simulink model "FinalProjectSimulinkModel_OBSTACLE"  (R2023b)
settings: Solver=VariableStepAuto  StartTime=0.0  StopTime=17  RelTol=1e-3
values from neighbouring files (symbols this model uses):
  dq_d_COM = [0.75; 0; 0; 0; 0; 0]    [FinalProject_init.m]
  dq_d_COM_Jump = [10; 0; 20; 0; -30; 0]    [FinalProject_init.m]
  dq_d_COM_Jump_2 = [12; 0; 21.2; 0; -35.6; 0]    [FinalProject_init.m]
  dtMPC = 0.03    [FinalProject_init.m]
  firstStairDist = 0.26    [FinalProject_init.m]
  flight_gait_2 = [tcrouch2;fFofft2;rFofft2;rlandt2;flandt2; tImpact]    [FinalProject_init.m]
  flight_gait_t = [tcrouch;fFofft;rFofft;rlandt;flandt; tImpact]    [FinalProject_init.m]
  kd_swing = 10    [FinalProject_init.m]
  kp_swing = 300    [FinalProject_init.m]
  kStep = 0.001    [FinalProject_init.m]
  NMPC = 10    [FinalProject_init.m]
  offsets = [0;tSwing;tSwing;0]    [FinalProject_init.m]
  q_d_crouch = [q_hip_roll_f ... (first row only)    [FinalProject_init.m]
  q_d_impact = [q_hip_roll_i_f ... (first row only)    [FinalProject_init.m]
  q_d_stand = [q_hip_roll_i;q_hip_pitch_i;q_knee_i]    [FinalProject_init.m]
  q_hip_roll_i = 0    [FinalProject_init.m]
  Qmpc = diag([100 100 50 1000 1000 500 4 4 4 1 1 1 0])    [FinalProject_init.m]
  rFofft = 0.12+tcrouch    (= 1.12)    [FinalProject_init.m]
  rFofft2 = 0.12+tcrouch2    (= 1.42)    [FinalProject_init.m]
  Rmpc = 0.00001*eye(12)    [FinalProject_init.m]
  task = 6    [FinalProject_init.m]
  tcrouch = 1.0    (= 1)    [FinalProject_init.m]
  tcrouch2 = 1.3    [FinalProject_init.m]
  tCycle = 0.3    [FinalProject_init.m]
  tRamp = 0.5    [FinalProject_init.m]
  tRamp_Jump = 0.05    [FinalProject_init.m]
  tRamp_Jump2 = 0.08    [FinalProject_init.m]
  tSlow = 0.3    [FinalProject_init.m]
  tSwing = tCycle/2    (= 0.15)    [FinalProject_init.m]
  x0_Trunk = [0;0;z_trunk_i-.15; 0;-0.271;0]    [FinalProject_init.m]
undefined symbols (not defined in the file or in its folder): kStepTheta, X, Y, Z
libraries: sm_lib x199, nesl_utility x53
(part 2 of 6)

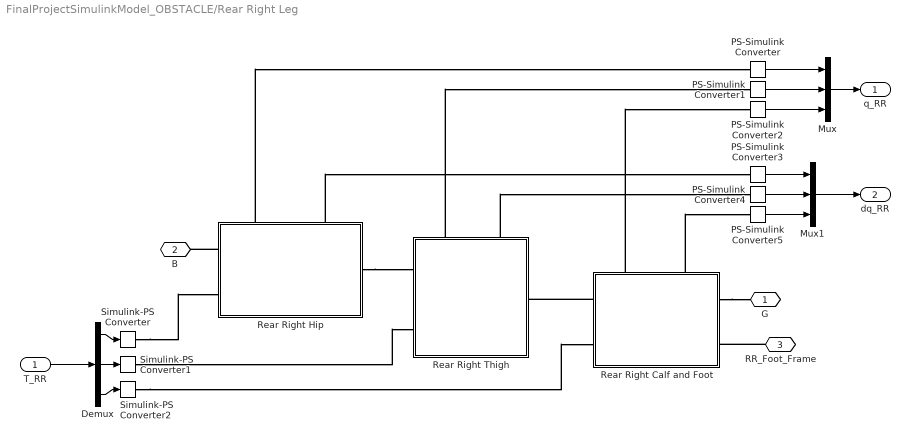
== system FinalProjectSimulinkModel_OBSTACLE/Rear Right Leg ==
  T_RR : Inport
  Demux : Demux  Outputs=3
  Mux : Mux  Inputs=3
  Mux1 : Mux  Inputs=3
  PS-Simulink Converter{,1..5} (6 alike) : nesl_utility/PS-Simulink Converter  PhysicalDomain=network_engine_domain  SubClassName=ps_output  LeftPortType=input  RightPortType=output  PseudoPeriodic=off  Frequencies=[]  VectorFormat=inherit  Unit=inherit  AffineConversion=off
  Rear Right Hip : Subsystem
      settings: PortSchema="{\"entries\":[{\"content\":{\"sides\":[{\"content\":{\"connectorIds\":[\"LConn1\",\"LConn2\"]},\"type\":\"ConnectorPlacement.EquallySpacedRectSide\",\"uuid\":\"d53fc21f-a4e5-460f-be2d-383a76a109ad\"},{\"content\":{\"connectorIds\":[\"RConn1\"],\"side\":\"RIGHT\"},\"type\":\"ConnectorPlacement.EquallySpacedRectSide\",\"uuid\":\"4a22f7e2-1f22-4597-903e-3f257006dede\"},{\"content\":{\"connectorIds\":[\"LConn3\",\"LConn4\"],\"side\":\"TOP\"},\"type\":\"ConnectorPlacement.EquallySpacedRectSide\",\"uuid\":\"7ea439a1-197b-4788-b0d2-cace68ebb6cf\"}]},\"type\":\"ConnectorPlacement.EquallySpacedConnector\",\"uuid\":\"bb801113-64bf-4d16-9167-4042132993b1\"}],\"packageUris\":[\"http://schema.mathworks.com/mf0/Connector/R2020b\"],\"version\":\"1.0\"}"
  Rear Right Thigh : Subsystem
      settings: PortSchema="{\"entries\":[{\"content\":{\"sides\":[{\"content\":{\"connectorIds\":[\"LConn1\",\"LConn2\"]},\"type\":\"ConnectorPlacement.EquallySpacedRectSide\",\"uuid\":\"d53fc21f-a4e5-460f-be2d-383a76a109ad\"},{\"content\":{\"connectorIds\":[\"RConn1\"],\"side\":\"RIGHT\"},\"type\":\"ConnectorPlacement.EquallySpacedRectSide\",\"uuid\":\"4a22f7e2-1f22-4597-903e-3f257006dede\"},{\"content\":{\"connectorIds\":[\"LConn3\",\"LConn4\"],\"side\":\"TOP\"},\"type\":\"ConnectorPlacement.EquallySpacedRectSide\",\"uuid\":\"7ea439a1-197b-4788-b0d2-cace68ebb6cf\"}]},\"type\":\"ConnectorPlacement.EquallySpacedConnector\",\"uuid\":\"bb801113-64bf-4d16-9167-4042132993b1\"}],\"packageUris\":[\"http://schema.mathworks.com/mf0/Connector/R2020b\"],\"version\":\"1.0\"}"
  Rear Right Calf and Foot : Subsystem
      settings: PortSchema="{\"entries\":[{\"content\":{\"sides\":[{\"content\":{\"connectorIds\":[\"LConn1\",\"LConn2\"]},\"type\":\"ConnectorPlacement.EquallySpacedRectSide\",\"uuid\":\"d53fc21f-a4e5-460f-be2d-383a76a109ad\"},{\"content\":{\"connectorIds\":[\"RConn1\",\"RConn2\"],\"side\":\"RIGHT\"},\"type\":\"ConnectorPlacement.EquallySpacedRectSide\",\"uuid\":\"4a22f7e2-1f22-4597-903e-3f257006dede\"},{\"content\":{\"connectorIds\":[\"LConn3\",\"LConn4\"],\"side\":\"TOP\"},\"type\":\"ConnectorPlacement.EquallySpacedRectSide\",\"uuid\":\"7ea439a1-197b-4788-b0d2-cace68ebb6cf\"}]},\"type\":\"ConnectorPlacement.EquallySpacedConnector\",\"uuid\":\"bb801113-64bf-4d16-9167-4042132993b1\"}],\"packageUris\":[\"http://schema.mathworks.com/mf0/Connector/R2020b\"],\"version\":\"1.0\"}"
  Simulink-PS Converter : nesl_utility/Simulink-PS Converter  PhysicalDomain=network_engine_domain  SubClassName=ps_input  LeftPortType=input  RightPortType=output  PseudoPeriodic=off  Frequencies=[]  NoiseDistribution=none  NoiseParameters=[]  Unit=1  AffineConversion=off  FilteringAndDerivatives=provide  SimscapeFilterOrder=1  InputFilterTimeConstant=0.001  UdotUserProvided=0
  Simulink-PS Converter1 : nesl_utility/Simulink-PS Converter  PhysicalDomain=network_engine_domain  SubClassName=ps_input  LeftPortType=input  RightPortType=output  PseudoPeriodic=off  Frequencies=[]  NoiseDistribution=none  NoiseParameters=[]  Unit=1  AffineConversion=off  FilteringAndDerivatives=provide  SimscapeFilterOrder=1  InputFilterTimeConstant=0.001  UdotUserProvided=0
  Simulink-PS Converter2 : nesl_utility/Simulink-PS Converter  PhysicalDomain=network_engine_domain  SubClassName=ps_input  LeftPortType=input  RightPortType=output  PseudoPeriodic=off  Frequencies=[]  NoiseDistribution=none  NoiseParameters=[]  Unit=1  AffineConversion=off  FilteringAndDerivatives=provide  SimscapeFilterOrder=1  InputFilterTimeConstant=0.001  UdotUserProvided=0
  G : PMIOPort  Side=Right
  B : PMIOPort  Port=2  Side=Left
  RR_Foot_Frame : PMIOPort  Port=3  Side=Right
  q_RR : Outport
  dq_RR : Outport  Port=2
  wires:
  T_RR/1 -> Demux/1
  Demux/2 -> Simulink-PS Converter1/1
  Demux/1 -> Simulink-PS Converter/1
  Demux/3 -> Simulink-PS Converter2/1
  PS-Simulink Converter/1 -> Mux/1
  PS-Simulink Converter1/1 -> Mux/2
  PS-Simulink Converter2/1 -> Mux/3
  PS-Simulink Converter4/1 -> Mux1/2
  PS-Simulink Converter5/1 -> Mux1/3
  PS-Simulink Converter3/1 -> Mux1/1
  Mux/1 -> q_RR/1
  Mux1/1 -> dq_RR/1
  connections:
  Rear Right Calf and Foot/LConn1 -- Rear Right Thigh/RConn1
  Rear Right Hip/RConn1 -- Rear Right Thigh/LConn1
  Rear Right Calf and Foot/RConn1 -- G/RConn1
  Rear Right Hip/LConn1 -- B/RConn1
  Simulink-PS Converter/RConn1 -- Rear Right Hip/LConn2
  Simulink-PS Converter1/RConn1 -- Rear Right Thigh/LConn2
  Simulink-PS Converter2/RConn1 -- Rear Right Calf and Foot/LConn2
  Rear Right Hip/LConn3 -- PS-Simulink Converter/LConn1
  Rear Right Thigh/LConn3 -- PS-Simulink Converter1/LConn1
  Rear Right Calf and Foot/LConn3 -- PS-Simulink Converter2/LConn1
  Rear Right Hip/LConn4 -- PS-Simulink Converter3/LConn1
  Rear Right Thigh/LConn4 -- PS-Simulink Converter4/LConn1
  Rear Right Calf and Foot/LConn4 -- PS-Simulink Converter5/LConn1
  RR_Foot_Frame/RConn1 -- Rear Right Calf and Foot/RConn2

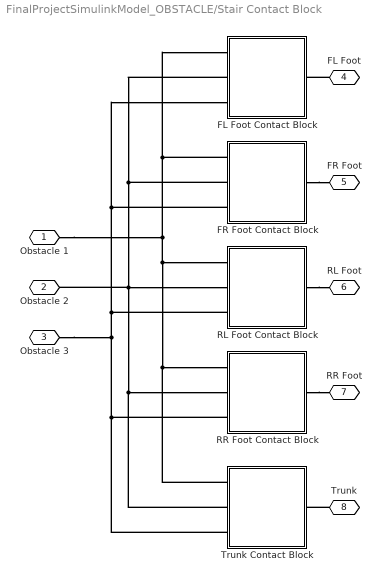
== system FinalProjectSimulinkModel_OBSTACLE/Stair Contact Block ==
  FL Foot Contact Block : Subsystem
  FR Foot Contact Block : Subsystem
  RL Foot Contact Block : Subsystem
  RR Foot Contact Block : Subsystem
  Trunk Contact Block : Subsystem
  Obstacle 1 : PMIOPort  Side=Left
  Obstacle 2 : PMIOPort  Port=2  Side=Left
  Obstacle 3 : PMIOPort  Port=3  Side=Left
  FL Foot : PMIOPort  Port=4  Side=Right
  FR Foot : PMIOPort  Port=5  Side=Right
  RL Foot : PMIOPort  Port=6  Side=Right
  RR Foot : PMIOPort  Port=7  Side=Right
  Trunk : PMIOPort  Port=8  Side=Right
  connections:
  Obstacle 1/RConn1 -- Trunk Contact Block/LConn1 -- RR Foot Contact Block/LConn1 -- RL Foot Contact Block/LConn1 -- FR Foot Contact Block/LConn1 -- FL Foot Contact Block/LConn1
  FL Foot Contact Block/LConn2 -- FR Foot Contact Block/LConn2 -- Trunk Contact Block/LConn2 -- RR Foot Contact Block/LConn2 -- Obstacle 2/RConn1 -- RL Foot Contact Block/LConn2
  Obstacle 3/RConn1 -- FR Foot Contact Block/LConn3 -- FL Foot Contact Block/LConn3 -- RL Foot Contact Block/LConn3 -- Trunk Contact Block/LConn3 -- RR Foot Contact Block/LConn3
  FR Foot Contact Block/RConn1 -- FR Foot/RConn1
  FL Foot/RConn1 -- FL Foot Contact Block/RConn1
  RL Foot Contact Block/RConn1 -- RL Foot/RConn1
  RR Foot Contact Block/RConn1 -- RR Foot/RConn1
  Trunk/RConn1 -- Trunk Contact Block/RConn1

== system FinalProjectSimulinkModel_OBSTACLE/base ==
  ReferenceFrame : sm_lib/Frames and Transforms/Reference Frame
  Visual : sm_lib/Body Elements/Brick Solid  GraphicAmbientColor=[0.15 0.15 0.15 1.0]  BasedOnType=Density  BrickDimensions=[0.001, 0.001, 0.001]  BrickDimensionsUnits=m  CenterOfMass=[0, 0, 0]  CenterOfMassUnits=m  GraphicDiffuseColor=[0.5, 0.5, 0.5]  Density=1000  DensityUnits=kg/m^3  DoExposeReferenceFrame=on  GraphicEmissiveColor=[0.0 0.0 0.0 1.0]  ExportEntireGeometry=off  SerializedFrames=<Frames/>  MarkerShape=Sphere  MarkerSize=10  GraphicType=FromGeometry  InertiaType=Custom  Mass=0  MassUnits=kg  MomentsOfInertia=[0, 0, 0]  MomentsOfInertiaUnits=kg*m^2  GraphicOpacity=1  ProductsOfInertia=[0, 0, 0]  ProductsOfInertiaUnits=kg*m^2  GraphicShininess=75  GraphicSpecularColor=[0.5 0.5 0.5 1.0]  GraphicVisPropType=SimpleVisualProperties
  VisualOriginTransform : sm_lib/Frames and Transforms/Rigid Transform  TranslationMethod=Cartesian  TranslationStandardOffset=0  TranslationStandardOffsetUnits=m  TranslationStandardAxis=+Z  TranslationCartesianOffset=[0, 0, 0]  TranslationCartesianOffsetUnits=m  TranslationROffset=0  TranslationROffsetUnits=m  TranslationZOffset=0  TranslationZOffsetUnits=m  TranslationThetaOffset=0  TranslationThetaOffsetUnits=deg  RotationMethod=RotationSequence  RotationAngleUnits=deg  RotationStandardAxis=+Z  RotationAngle=0.0  RotationArbitraryAxis=[0 0 1]  FollAlignAxisA=+X  BaseAlignAxisA=+Y  FollAlignAxisB=+Y  BaseAlignAxisB=+Z  RotationSequenceAxes=BaseAxes  RotationSequence=XYZ  RotationSequenceAngles=[0, 0, 0]  RotationSequenceAnglesUnits=rad  RotationMatrix=[1 0 0; 0 1 0; 0 0 1]  Quaternion=[1 0 0 0]
  floating_base_OriginTransform : sm_lib/Frames and Transforms/Rigid Transform  TranslationMethod=Cartesian  TranslationStandardOffset=0  TranslationStandardOffsetUnits=m  TranslationStandardAxis=+Z  TranslationCartesianOffset=[0, 0, 0]  TranslationCartesianOffsetUnits=m  TranslationROffset=0  TranslationROffsetUnits=m  TranslationZOffset=0  TranslationZOffsetUnits=m  TranslationThetaOffset=0  TranslationThetaOffsetUnits=deg  RotationMethod=RotationSequence  RotationAngleUnits=deg  RotationStandardAxis=+Z  RotationAngle=0.0  RotationArbitraryAxis=[0 0 1]  FollAlignAxisA=+X  BaseAlignAxisA=+Y  FollAlignAxisB=+Y  BaseAlignAxisB=+Z  RotationSequenceAxes=BaseAxes  RotationSequence=XYZ  RotationSequenceAngles=[0, 0, 0]  RotationSequenceAnglesUnits=rad  RotationMatrix=[1 0 0; 0 1 0; 0 0 1]  Quaternion=[1 0 0 0]
  F : PMIOPort  Side=Left
  F1 : PMIOPort  Port=2  Side=Right
  connections:
  VisualOriginTransform/LConn1 -- ReferenceFrame/RConn1 -- F/RConn1 -- floating_base_OriginTransform/LConn1
  Visual/RConn1 -- VisualOriginTransform/RConn1
  floating_base_OriginTransform/RConn1 -- F1/RConn1

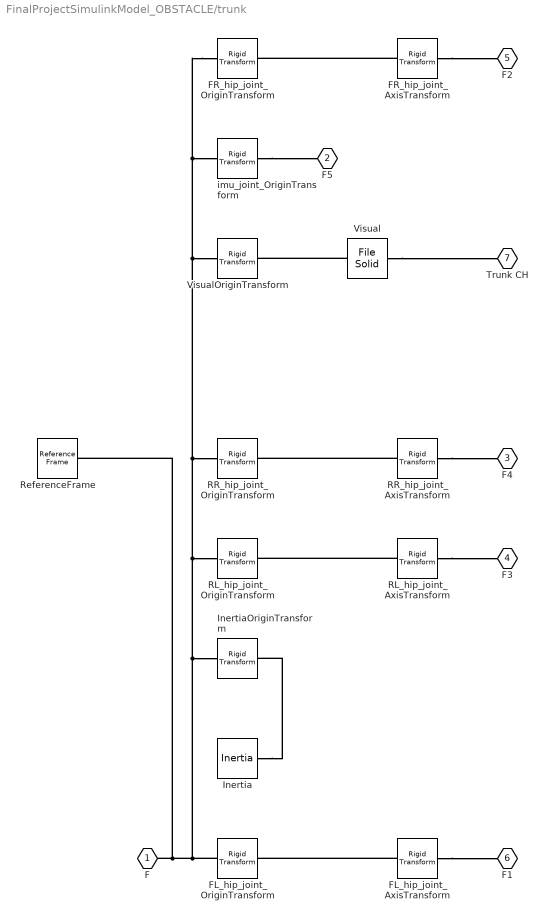
== system FinalProjectSimulinkModel_OBSTACLE/trunk ==
  FL_hip_joint_AxisTransform : sm_lib/Frames and Transforms/Rigid Transform  TranslationMethod=Cartesian  TranslationStandardOffset=0  TranslationStandardOffsetUnits=m  TranslationStandardAxis=+Z  TranslationCartesianOffset=[0, 0, 0]  TranslationCartesianOffsetUnits=m  TranslationROffset=0  TranslationROffsetUnits=m  TranslationZOffset=0  TranslationZOffsetUnits=m  TranslationThetaOffset=0  TranslationThetaOffsetUnits=deg  RotationMethod=ArbitraryAxis  RotationAngleUnits=rad  RotationStandardAxis=+Z  RotationAngle=1.570796326794897  RotationArbitraryAxis=[-0, 1, 0]  FollAlignAxisA=+X  BaseAlignAxisA=+Y  FollAlignAxisB=+Y  BaseAlignAxisB=+Z  RotationSequenceAxes=FollowerAxes  RotationSequence=XYX  RotationSequenceAngles=[0 0 0]  RotationSequenceAnglesUnits=deg  RotationMatrix=[1 0 0; 0 1 0; 0 0 1]  Quaternion=[1 0 0 0]
  FL_hip_joint_OriginTransform : sm_lib/Frames and Transforms/Rigid Transform  TranslationMethod=Cartesian  TranslationStandardOffset=0  TranslationStandardOffsetUnits=m  TranslationStandardAxis=+Z  TranslationCartesianOffset=[0.1805, 0.047, 0]  TranslationCartesianOffsetUnits=m  TranslationROffset=0  TranslationROffsetUnits=m  TranslationZOffset=0  TranslationZOffsetUnits=m  TranslationThetaOffset=0  TranslationThetaOffsetUnits=deg  RotationMethod=RotationSequence  RotationAngleUnits=deg  RotationStandardAxis=+Z  RotationAngle=0.0  RotationArbitraryAxis=[0 0 1]  FollAlignAxisA=+X  BaseAlignAxisA=+Y  FollAlignAxisB=+Y  BaseAlignAxisB=+Z  RotationSequenceAxes=BaseAxes  RotationSequence=XYZ  RotationSequenceAngles=[0, 0, 0]  RotationSequenceAnglesUnits=rad  RotationMatrix=[1 0 0; 0 1 0; 0 0 1]  Quaternion=[1 0 0 0]
  FR_hip_joint_AxisTransform : sm_lib/Frames and Transforms/Rigid Transform  TranslationMethod=Cartesian  TranslationStandardOffset=0  TranslationStandardOffsetUnits=m  TranslationStandardAxis=+Z  TranslationCartesianOffset=[0, 0, 0]  TranslationCartesianOffsetUnits=m  TranslationROffset=0  TranslationROffsetUnits=m  TranslationZOffset=0  TranslationZOffsetUnits=m  TranslationThetaOffset=0  TranslationThetaOffsetUnits=deg  RotationMethod=ArbitraryAxis  RotationAngleUnits=rad  RotationStandardAxis=+Z  RotationAngle=1.570796326794897  RotationArbitraryAxis=[-0, 1, 0]  FollAlignAxisA=+X  BaseAlignAxisA=+Y  FollAlignAxisB=+Y  BaseAlignAxisB=+Z  RotationSequenceAxes=FollowerAxes  RotationSequence=XYX  RotationSequenceAngles=[0 0 0]  RotationSequenceAnglesUnits=deg  RotationMatrix=[1 0 0; 0 1 0; 0 0 1]  Quaternion=[1 0 0 0]
  FR_hip_joint_OriginTransform : sm_lib/Frames and Transforms/Rigid Transform  TranslationMethod=Cartesian  TranslationStandardOffset=0  TranslationStandardOffsetUnits=m  TranslationStandardAxis=+Z  TranslationCartesianOffset=[0.1805, -0.047, 0]  TranslationCartesianOffsetUnits=m  TranslationROffset=0  TranslationROffsetUnits=m  TranslationZOffset=0  TranslationZOffsetUnits=m  TranslationThetaOffset=0  TranslationThetaOffsetUnits=deg  RotationMethod=RotationSequence  RotationAngleUnits=deg  RotationStandardAxis=+Z  RotationAngle=0.0  RotationArbitraryAxis=[0 0 1]  FollAlignAxisA=+X  BaseAlignAxisA=+Y  FollAlignAxisB=+Y  BaseAlignAxisB=+Z  RotationSequenceAxes=BaseAxes  RotationSequence=XYZ  RotationSequenceAngles=[0, 0, 0]  RotationSequenceAnglesUnits=rad  RotationMatrix=[1 0 0; 0 1 0; 0 0 1]  Quaternion=[1 0 0 0]
  Inertia : sm_lib/Body Elements/Inertia  InertiaType=Custom  Mass=6  MassUnits=kg  CenterOfMass=[0, 0, 0]  CenterOfMassUnits=m  MomentsOfInertia=[0.0158533, 0.0377999, 0.0456542]  MomentsOfInertiaUnits=kg*m^2  ProductsOfInertia=[-2.75e-05, -6.109999999999999e-05, -3.66e-05]  ProductsOfInertiaUnits=kg*m^2  GraphicType=None  MarkerShape=Inertia  MarkerSize=20  GraphicVisPropType=SimpleVisualProperties  GraphicDiffuseColor=[0.5 0.5 0.5]  GraphicSpecularColor=[0.5 0.5 0.5 1.0]  GraphicAmbientColor=[0.15 0.15 0.15 1.0]  GraphicEmissiveColor=[0.0 0.0 0.0 1.0]  GraphicShininess=75  GraphicOpacity=1.0
  InertiaOriginTransform : sm_lib/Frames and Transforms/Rigid Transform  TranslationMethod=Cartesian  TranslationStandardOffset=0  TranslationStandardOffsetUnits=m  TranslationStandardAxis=+Z  TranslationCartesianOffset=[0, 0.0041, -0.0005]  TranslationCartesianOffsetUnits=m  TranslationROffset=0  TranslationROffsetUnits=m  TranslationZOffset=0  TranslationZOffsetUnits=m  TranslationThetaOffset=0  TranslationThetaOffsetUnits=deg  RotationMethod=RotationSequence  RotationAngleUnits=deg  RotationStandardAxis=+Z  RotationAngle=0.0  RotationArbitraryAxis=[0 0 1]  FollAlignAxisA=+X  BaseAlignAxisA=+Y  FollAlignAxisB=+Y  BaseAlignAxisB=+Z  RotationSequenceAxes=BaseAxes  RotationSequence=XYZ  RotationSequenceAngles=[0, 0, 0]  RotationSequenceAnglesUnits=rad  RotationMatrix=[1 0 0; 0 1 0; 0 0 1]  Quaternion=[1 0 0 0]
  RL_hip_joint_AxisTransform : sm_lib/Frames and Transforms/Rigid Transform  TranslationMethod=Cartesian  TranslationStandardOffset=0  TranslationStandardOffsetUnits=m  TranslationStandardAxis=+Z  TranslationCartesianOffset=[0, 0, 0]  TranslationCartesianOffsetUnits=m  TranslationROffset=0  TranslationROffsetUnits=m  TranslationZOffset=0  TranslationZOffsetUnits=m  TranslationThetaOffset=0  TranslationThetaOffsetUnits=deg  RotationMethod=ArbitraryAxis  RotationAngleUnits=rad  RotationStandardAxis=+Z  RotationAngle=1.570796326794897  RotationArbitraryAxis=[-0, 1, 0]  FollAlignAxisA=+X  BaseAlignAxisA=+Y  FollAlignAxisB=+Y  BaseAlignAxisB=+Z  RotationSequenceAxes=FollowerAxes  RotationSequence=XYX  RotationSequenceAngles=[0 0 0]  RotationSequenceAnglesUnits=deg  RotationMatrix=[1 0 0; 0 1 0; 0 0 1]  Quaternion=[1 0 0 0]
  RL_hip_joint_OriginTransform : sm_lib/Frames and Transforms/Rigid Transform  TranslationMethod=Cartesian  TranslationStandardOffset=0  TranslationStandardOffsetUnits=m  TranslationStandardAxis=+Z  TranslationCartesianOffset=[-0.1805, 0.047, 0]  TranslationCartesianOffsetUnits=m  TranslationROffset=0  TranslationROffsetUnits=m  TranslationZOffset=0  TranslationZOffsetUnits=m  TranslationThetaOffset=0  TranslationThetaOffsetUnits=deg  RotationMethod=RotationSequence  RotationAngleUnits=deg  RotationStandardAxis=+Z  RotationAngle=0.0  RotationArbitraryAxis=[0 0 1]  FollAlignAxisA=+X  BaseAlignAxisA=+Y  FollAlignAxisB=+Y  BaseAlignAxisB=+Z  RotationSequenceAxes=BaseAxes  RotationSequence=XYZ  RotationSequenceAngles=[0, 0, 0]  RotationSequenceAnglesUnits=rad  RotationMatrix=[1 0 0; 0 1 0; 0 0 1]  Quaternion=[1 0 0 0]
  RR_hip_joint_AxisTransform : sm_lib/Frames and Transforms/Rigid Transform  TranslationMethod=Cartesian  TranslationStandardOffset=0  TranslationStandardOffsetUnits=m  TranslationStandardAxis=+Z  TranslationCartesianOffset=[0, 0, 0]  TranslationCartesianOffsetUnits=m  TranslationROffset=0  TranslationROffsetUnits=m  TranslationZOffset=0  TranslationZOffsetUnits=m  TranslationThetaOffset=0  TranslationThetaOffsetUnits=deg  RotationMethod=ArbitraryAxis  RotationAngleUnits=rad  RotationStandardAxis=+Z  RotationAngle=1.570796326794897  RotationArbitraryAxis=[-0, 1, 0]  FollAlignAxisA=+X  BaseAlignAxisA=+Y  FollAlignAxisB=+Y  BaseAlignAxisB=+Z  RotationSequenceAxes=FollowerAxes  RotationSequence=XYX  RotationSequenceAngles=[0 0 0]  RotationSequenceAnglesUnits=deg  RotationMatrix=[1 0 0; 0 1 0; 0 0 1]  Quaternion=[1 0 0 0]
  RR_hip_joint_OriginTransform : sm_lib/Frames and Transforms/Rigid Transform  TranslationMethod=Cartesian  TranslationStandardOffset=0  TranslationStandardOffsetUnits=m  TranslationStandardAxis=+Z  TranslationCartesianOffset=[-0.1805, -0.047, 0]  TranslationCartesianOffsetUnits=m  TranslationROffset=0  TranslationROffsetUnits=m  TranslationZOffset=0  TranslationZOffsetUnits=m  TranslationThetaOffset=0  TranslationThetaOffsetUnits=deg  RotationMethod=RotationSequence  RotationAngleUnits=deg  RotationStandardAxis=+Z  RotationAngle=0.0  RotationArbitraryAxis=[0 0 1]  FollAlignAxisA=+X  BaseAlignAxisA=+Y  FollAlignAxisB=+Y  BaseAlignAxisB=+Z  RotationSequenceAxes=BaseAxes  RotationSequence=XYZ  RotationSequenceAngles=[0, 0, 0]  RotationSequenceAnglesUnits=rad  RotationMatrix=[1 0 0; 0 1 0; 0 0 1]  Quaternion=[1 0 0 0]
  ReferenceFrame : sm_lib/Frames and Transforms/Reference Frame
  Visual : sm_lib/Body Elements/File Solid  ExtGeomFileName=a1_description/meshes/trunk.stl  UnitType=Custom  ExtGeomFileUnits=m  StepReaderType=HEX  ExportConvexHullGeometry=on  InertiaType=Custom  Mass=0  MassUnits=kg  CenterOfMass=[0, 0, 0]  CenterOfMassUnits=m  MomentsOfInertia=[0, 0, 0]  MomentsOfInertiaUnits=kg*m^2  ProductsOfInertia=[0, 0, 0]  ProductsOfInertiaUnits=kg*m^2  BasedOnType=DensityFromFile  Density=1000  DensityUnits=kg/m^3  DoExposeReferenceFrame=on  SerializedFrames=<Frames/>  GraphicType=FromGeometry  MarkerShape=Sphere  MarkerSize=10  GraphicVisPropType=SimpleVisualProperties  GraphicDiffuseColor=[0.2 0.2 0.2]  GraphicSpecularColor=[0.5 0.5 0.5 1.0]  GraphicAmbientColor=[0.15 0.15 0.15 1.0]  GraphicEmissiveColor=[0.0 0.0 0.0 1.0]  GraphicShininess=75  GraphicOpacity=1
  VisualOriginTransform : sm_lib/Frames and Transforms/Rigid Transform  TranslationMethod=Cartesian  TranslationStandardOffset=0  TranslationStandardOffsetUnits=m  TranslationStandardAxis=+Z  TranslationCartesianOffset=[0, 0, 0]  TranslationCartesianOffsetUnits=m  TranslationROffset=0  TranslationROffsetUnits=m  TranslationZOffset=0  TranslationZOffsetUnits=m  TranslationThetaOffset=0  TranslationThetaOffsetUnits=deg  RotationMethod=RotationSequence  RotationAngleUnits=deg  RotationStandardAxis=+Z  RotationAngle=0.0  RotationArbitraryAxis=[0 0 1]  FollAlignAxisA=+X  BaseAlignAxisA=+Y  FollAlignAxisB=+Y  BaseAlignAxisB=+Z  RotationSequenceAxes=BaseAxes  RotationSequence=XYZ  RotationSequenceAngles=[0, 0, 0]  RotationSequenceAnglesUnits=rad  RotationMatrix=[1 0 0; 0 1 0; 0 0 1]  Quaternion=[1 0 0 0]
  imu_joint_OriginTransform : sm_lib/Frames and Transforms/Rigid Transform  TranslationMethod=Cartesian  TranslationStandardOffset=0  TranslationStandardOffsetUnits=m  TranslationStandardAxis=+Z  TranslationCartesianOffset=[0, 0, 0]  TranslationCartesianOffsetUnits=m  TranslationROffset=0  TranslationROffsetUnits=m  TranslationZOffset=0  TranslationZOffsetUnits=m  TranslationThetaOffset=0  TranslationThetaOffsetUnits=deg  RotationMethod=RotationSequence  RotationAngleUnits=deg  RotationStandardAxis=+Z  RotationAngle=0.0  RotationArbitraryAxis=[0 0 1]  FollAlignAxisA=+X  BaseAlignAxisA=+Y  FollAlignAxisB=+Y  BaseAlignAxisB=+Z  RotationSequenceAxes=BaseAxes  RotationSequence=XYZ  RotationSequenceAngles=[0, 0, 0]  RotationSequenceAnglesUnits=rad  RotationMatrix=[1 0 0; 0 1 0; 0 0 1]  Quaternion=[1 0 0 0]
  F : PMIOPort  Side=Left
  F5 : PMIOPort  Port=2  Side=Right
  F4 : PMIOPort  Port=3  Side=Right
  F3 : PMIOPort  Port=4  Side=Right
  F2 : PMIOPort  Port=5  Side=Right
  F1 : PMIOPort  Port=6  Side=Right
  Trunk CH : PMIOPort  Port=7  Side=Right
  connections:
  FL_hip_joint_AxisTransform/RConn1 -- F1/RConn1
  FL_hip_joint_AxisTransform/LConn1 -- FL_hip_joint_OriginTransform/RConn1
  FR_hip_joint_AxisTransform/RConn1 -- F2/RConn1
  FR_hip_joint_AxisTransform/LConn1 -- FR_hip_joint_OriginTransform/RConn1
  Inertia/RConn1 -- InertiaOriginTransform/RConn1
  RL_hip_joint_AxisTransform/RConn1 -- F3/RConn1
  RL_hip_joint_AxisTransform/LConn1 -- RL_hip_joint_OriginTransform/RConn1
  RR_hip_joint_AxisTransform/RConn1 -- F4/RConn1
  RR_hip_joint_AxisTransform/LConn1 -- RR_hip_joint_OriginTransform/RConn1
  FR_hip_joint_OriginTransform/LConn1 -- FL_hip_joint_OriginTransform/LConn1 -- ReferenceFrame/RConn1 -- F/RConn1 -- InertiaOriginTransform/LConn1 -- RL_hip_joint_OriginTransform/LConn1 -- RR_hip_joint_OriginTransform/LConn1 -- VisualOriginTransform/LConn1 -- imu_joint_OriginTransform/LConn1
  Visual/RConn1 -- VisualOriginTransform/RConn1
  imu_joint_OriginTransform/RConn1 -- F5/RConn1
  Visual/LConn1 -- Trunk CH/RConn1

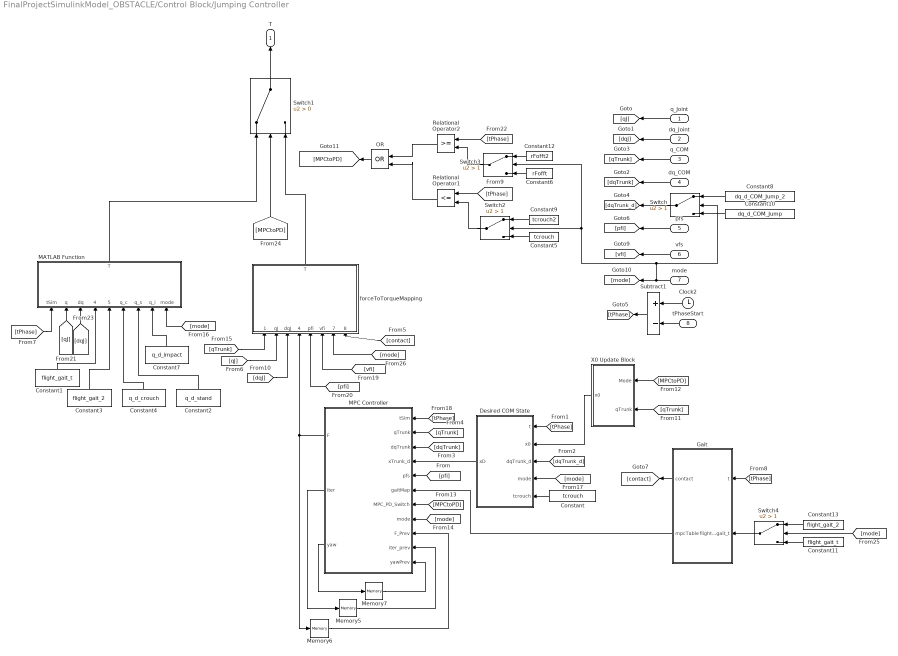
== system FinalProjectSimulinkModel_OBSTACLE/Control Block/Jumping Controller ==
  q_Joint : Inport
  dq_Joint : Inport  Port=2
  q_COM : Inport  Port=3
  dq_COM : Inport  Port=4
  pfs : Inport  Port=5
  vfs : Inport  Port=6
  mode : Inport  Port=7
  tPhaseStart : Inport  Port=8
  Clock2 : Clock
  Constant : Constant  Value=tcrouch
  Constant1 : Constant  Value=flight_gait_t
  Constant10 : Constant  Value=dq_d_COM_Jump
  Constant11 : Constant  Value=flight_gait_t
  Constant12 : Constant  Value=rFofft2
  Constant13 : Constant  Value=flight_gait_2
  Constant2 : Constant  Value=q_d_stand
  Constant3 : Constant  Value=flight_gait_2
  Constant4 : Constant  Value=q_d_crouch
  Constant5 : Constant  Value=tcrouch
  Constant6 : Constant  Value=rFofft
  Constant7 : Constant  Value=q_d_impact
  Constant8 : Constant  Value=dq_d_COM_Jump_2
  Constant9 : Constant  Value=tcrouch2
  Desired COM State : MATLAB Function  TreatAsAtomicUnit=on
  Gait : MATLAB Function  TreatAsAtomicUnit=on
  MATLAB Function : MATLAB Function  TreatAsAtomicUnit=on
  MPC Controller : MATLAB Function  TreatAsAtomicUnit=on
  Memory5 : Memory  InitialCondition=-1
  Memory6 : Memory  InitialCondition=ones(12,1)*0.0001
  Memory7 : Memory
  OR : Logic  Operator=OR  IconShape=distinctive  AllPortsSameDT=off  OutDataTypeStr=boolean
  Relational Operator1 : RelationalOperator  Operator=<=  OutDataTypeStr=boolean  RndMeth=Simplest  InputSameDT=off
  Relational Operator2 : RelationalOperator  OutDataTypeStr=boolean  RndMeth=Simplest  InputSameDT=off
  Subtract1 : Sum  Inputs=+-
  Switch{,2..4} (4 alike) : Switch  Criteria=u2 > Threshold  Threshold=1  SaturateOnIntegerOverflow=off  InputSameDT=off
  Switch1 : Switch  Criteria=u2 > Threshold  SaturateOnIntegerOverflow=off  InputSameDT=off
  X0 Update Block : Subsystem
  forceToTorqueMapping : MATLAB Function  TreatAsAtomicUnit=on
  T : Outport
  wires:
  pfs/1 -> [pfi]
  q_COM/1 -> [qTrunk]
  dq_COM/1 -> [dqTrunk]
  vfs/1 -> [vfi]
  q_Joint/1 -> [qJ]
  dq_Joint/1 -> [dqJ]
  Clock2/1 -> Subtract1/1
  Subtract1/1 -> [tPhase]
  tPhaseStart/1 -> Subtract1/2
  [tPhase] -> Relational Operator2/1
  OR/1 -> [MPCtoPD]
  Gait/1(contact) -> [contact]
  Switch1/1 -> T/1
  [tPhase] -> MATLAB Function/1(tSim)
  forceToTorqueMapping/1(T) -> Switch1/3
  Relational Operator1/1 -> OR/2
  Memory5/1 -> MPC Controller/10(iter_prev)
  [MPCtoPD] -> Switch1/2
  Gait/2(mpcTable) -> MPC Controller/6(gaitMap)
  Memory7/1 -> MPC Controller/11(yawPrev)
  Desired COM State/1(xD) -> MPC Controller/4(xTrunk_d)
  MPC Controller/1(F) -> Memory6/1, forceToTorqueMapping/4(F_SRBD)
  [qJ] -> MATLAB Function/2(q)
  [qTrunk] -> forceToTorqueMapping/1(qTrunk)
  [contact] -> forceToTorqueMapping/8(contact)
  [tPhase] -> Desired COM State/1(t)
  [pfi] -> MPC Controller/5(pfs)
  [dqTrunk_d] -> Desired COM State/3(dqTrunk_d)
  Constant/1 -> Desired COM State/5(tcrouch)
  Memory6/1 -> MPC Controller/9(F_Prev)
  [MPCtoPD] -> X0 Update Block/1(Mode)
  [qTrunk] -> X0 Update Block/2(qTrunk)
  Constant1/1 -> MATLAB Function/4(flight_gait_1)
  Constant2/1 -> MATLAB Function/7(q_s)
  [dqTrunk] -> MPC Controller/3(dqTrunk)
  [dqJ] -> MATLAB Function/3(dq)
  MPC Controller/2(iter) -> Memory5/1
  [MPCtoPD] -> MPC Controller/7(MPC_PD_Switch)
  [qJ] -> forceToTorqueMapping/2(qJ)
  [qTrunk] -> MPC Controller/2(qTrunk)
  MATLAB Function/1(T) -> Switch1/1
  Relational Operator2/1 -> OR/1
  Constant4/1 -> MATLAB Function/6(q_c)
  MPC Controller/3(yaw) -> Memory7/1
  [tPhase] -> Relational Operator1/1
  X0 Update Block/1(x0) -> Desired COM State/2(x0)
  [tPhase] -> MPC Controller/1(tSim)
  [tPhase] -> Gait/1(t)
  [mode] -> MPC Controller/8(mode)
  [mode] -> MATLAB Function/9(mode)
  Constant3/1 -> MATLAB Function/5(flight_gait_2)
  Constant7/1 -> MATLAB Function/8(q_i)
  Constant8/1 -> Switch/1
  Constant10/1 -> Switch/3
  Switch/1 -> [dqTrunk_d]
  [mode] -> Desired COM State/4(mode)
  Constant5/1 -> Switch2/3
  Constant9/1 -> Switch2/1
  Switch2/1 -> Relational Operator1/2
  Switch3/1 -> Relational Operator2/2
  mode/1 -> Switch3/2, Switch2/2, Switch/2, [mode]
  Constant6/1 -> Switch3/3
  Constant12/1 -> Switch3/1
  [dqJ] -> forceToTorqueMapping/3(dqJ)
  [vfi] -> forceToTorqueMapping/6(vfi)
  [pfi] -> forceToTorqueMapping/5(pfi)
  [mode] -> Switch4/2
  Constant11/1 -> Switch4/3
  Constant13/1 -> Switch4/1
  Switch4/1 -> Gait/2(flight_gait_t)
  [mode] -> forceToTorqueMapping/7(mode)

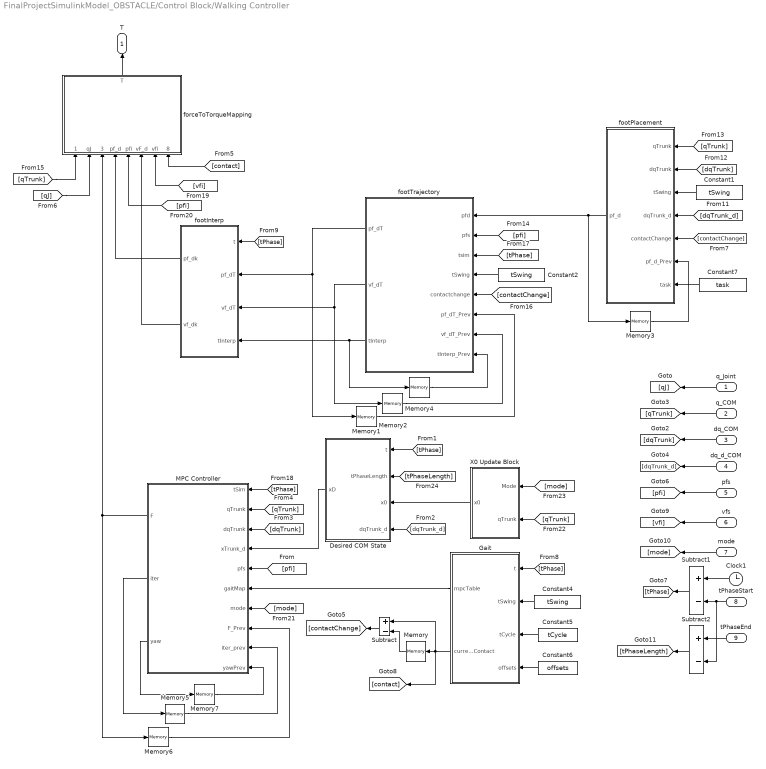
== system FinalProjectSimulinkModel_OBSTACLE/Control Block/Walking Controller ==
  q_Joint : Inport
  q_COM : Inport  Port=2
  dq_COM : Inport  Port=3
  dq_d_COM : Inport  Port=4
  pfs : Inport  Port=5
  vfs : Inport  Port=6
  mode : Inport  Port=7
  tPhaseStart : Inport  Port=8
  tPhaseEnd : Inport  Port=9
  Clock1 : Clock
  Constant1 : Constant  Value=tSwing
  Constant2 : Constant  Value=tSwing
  Constant4 : Constant  Value=tSwing
  Constant5 : Constant  Value=tCycle
  Constant6 : Constant  Value=offsets
  Constant7 : Constant  Value=task
  Desired COM State : MATLAB Function  TreatAsAtomicUnit=on
  Gait : MATLAB Function  TreatAsAtomicUnit=on
  MPC Controller : MATLAB Function  TreatAsAtomicUnit=on
  Memory : Memory  InitialCondition=[1;1;1;1]
  Memory1 : Memory  InitialCondition=zeros(100,12)
  Memory2 : Memory  InitialCondition=zeros(100,12)
  Memory3 : Memory  InitialCondition=zeros(12,1)
  Memory4 : Memory  InitialCondition=repmat(linspace(0,tCycle,100)',[1,4])
  Memory5 : Memory  InitialCondition=-1
  Memory6 : Memory  InitialCondition=ones(12,1)*0.0001
  Memory7 : Memory
  Subtract : Sum  Inputs=+-
  Subtract1 : Sum  Inputs=+-
  Subtract2 : Sum  Inputs=+-
  X0 Update Block : Subsystem
  footInterp : MATLAB Function  TreatAsAtomicUnit=on
  footPlacement : MATLAB Function  TreatAsAtomicUnit=on
  footTrajectory : MATLAB Function  TreatAsAtomicUnit=on
  forceToTorqueMapping : MATLAB Function  TreatAsAtomicUnit=on
  T : Outport
  wires:
  [vfi] -> forceToTorqueMapping/7(vfi)
  [tPhase] -> MPC Controller/1(tSim)
  [qJ] -> forceToTorqueMapping/2(qJ)
  Constant7/1 -> footPlacement/7(task)
  MPC Controller/1(F) -> Memory6/1, forceToTorqueMapping/3(F_SRBD)
  MPC Controller/2(iter) -> Memory5/1
  Memory1/1 -> footTrajectory/6(pf_dT_Prev)
  Memory2/1 -> footTrajectory/7(vf_dT_Prev)
  footInterp/1(pf_dk) -> forceToTorqueMapping/4(pf_d)
  [tPhase] -> Desired COM State/1(t)
  Constant6/1 -> Gait/4(offsets)
  [tPhase] -> footInterp/1(t)
  Memory7/1 -> MPC Controller/10(yawPrev)
  [tPhase] -> footTrajectory/3(tsim)
  [dqTrunk_d] -> footPlacement/4(dqTrunk_d)
  Constant5/1 -> Gait/3(tCycle)
  [qTrunk] -> MPC Controller/2(qTrunk)
  [dqTrunk] -> footPlacement/2(dqTrunk)
  [pfi] -> forceToTorqueMapping/5(pfi)
  Gait/1(mpcTable) -> MPC Controller/6(gaitMap)
  footPlacement/1(pf_d) -> Memory3/1, footTrajectory/1(pfd)
  Subtract/1 -> [contactChange]
  forceToTorqueMapping/1(T) -> T/1
  footTrajectory/2(vf_dT) -> Memory2/1, footInterp/3(vf_dT)
  Memory3/1 -> footPlacement/6(pf_d_Prev)
  Gait/2(currentContact) -> Subtract/1, [contact], Memory/1
  [contactChange] -> footPlacement/5(contactChange)
  [contactChange] -> footTrajectory/5(contactchange)
  footInterp/2(vf_dk) -> forceToTorqueMapping/6(vF_d)
  footTrajectory/3(tInterp) -> Memory4/1, footInterp/4(tInterp)
  [qTrunk] -> footPlacement/1(qTrunk)
  Memory4/1 -> footTrajectory/8(tInterp_Prev)
  Constant1/1 -> footPlacement/3(tSwing)
  footTrajectory/1(pf_dT) -> Memory1/1, footInterp/2(pf_dT)
  [tPhase] -> Gait/1(t)
  [qTrunk] -> forceToTorqueMapping/1(qTrunk)
  Constant4/1 -> Gait/2(tSwing)
  MPC Controller/3(yaw) -> Memory7/1
  Desired COM State/1(xD) -> MPC Controller/4(xTrunk_d)
  [dqTrunk] -> MPC Controller/3(dqTrunk)
  Memory6/1 -> MPC Controller/8(F_Prev)
  Memory/1 -> Subtract/2
  Memory5/1 -> MPC Controller/9(iter_prev)
  Constant2/1 -> footTrajectory/4(tSwing)
  [pfi] -> MPC Controller/5(pfs)
  [pfi] -> footTrajectory/2(pfs)
  [contact] -> forceToTorqueMapping/8(contact)
  q_COM/1 -> [qTrunk]
  q_Joint/1 -> [qJ]
  pfs/1 -> [pfi]
  dq_d_COM/1 -> [dqTrunk_d]
  vfs/1 -> [vfi]
  dq_COM/1 -> [dqTrunk]
  mode/1 -> [mode]
  [mode] -> MPC Controller/7(mode)
  tPhaseStart/1 -> Subtract2/2, Subtract1/2
  Clock1/1 -> Subtract1/1
  Subtract1/1 -> [tPhase]
  [mode] -> X0 Update Block/1(Mode)
  [qTrunk] -> X0 Update Block/2(qTrunk)
  X0 Update Block/1(x0) -> Desired COM State/3(x0)
  [dqTrunk_d] -> Desired COM State/4(dqTrunk_d)
  tPhaseEnd/1 -> Subtract2/1
  Subtract2/1 -> [tPhaseLength]
  [tPhaseLength] -> Desired COM State/2(tPhaseLength)

== system FinalProjectSimulinkModel_OBSTACLE/Front Left Leg/Front Left Calf and Foot ==
  FL_calf : Subsystem
  FL_calf_joint : sm_lib/Joints/Revolute Joint  JointMode=Normal  SenseConstraintForce=off  SenseConstraintForceX=off  SenseConstraintForceY=off  SenseConstraintForceZ=off  SenseConstraintTorque=off  SenseConstraintTorqueX=off  SenseConstraintTorqueY=off  SenseConstraintTorqueZ=off  SenseTotalForce=off  SenseTotalForceX=off  SenseTotalForceY=off  SenseTotalForceZ=off  SenseTotalTorque=off  SenseTotalTorqueX=off  SenseTotalTorqueY=off  SenseTotalTorqueZ=off  CompositeWrenchDir=FollowerOnBase  CompositeWrenchFrame=BaseFrame  EquilibriumPosition=0  EquilibriumPositionUnits=deg  SpringStiffness=0  SpringStiffnessUnits=N*m/deg  DampingCoefficient=0.01  DampingCoefficientUnits=kg*m^2/(rad*s)  TorqueActuationMode=InputTorque  MotionActuationMode=ComputedMotion  SensePosition=on  SenseVelocity=on  SenseAcceleration=off  SenseTorqueForce=off  SenseLowerLimitTorqueForce=off  SenseUpperLimitTorqueForce=off  LowerLimitSpecify=on  LowerLimitBound=-2.69653369433  LowerLimitBoundUnits=rad  LowerLimitStiffness=1e4  LowerLimitStiffnessUnits=N*m/deg  LowerLimitDamping=10  LowerLimitDampingUnits=N*m/(deg/s)  LowerLimitTransitionRegionWidth=0.1  LowerLimitTransitionRegionWidthUnits=deg  UpperLimitSpecify=on  UpperLimitBound=-0.916297857297  UpperLimitBoundUnits=rad  UpperLimitStiffness=1e4  UpperLimitStiffnessUnits=N*m/deg  UpperLimitDamping=10  UpperLimitDampingUnits=N*m/(deg/s)  UpperLimitTransitionRegionWidth=0.1  UpperLimitTransitionRegionWidthUnits=deg  PositionTargetSpecify=on  PositionTargetPriority=High  PositionTargetValue=q_knee_i  PositionTargetValueUnits=rad  VelocityTargetSpecify=off  VelocityTargetPriority=High  VelocityTargetValue=0  VelocityTargetValueUnits=deg/s
  FL_foot : Subsystem
  FL_foot_fixed : sm_lib/Joints/Weld Joint  JointMode=Normal  SenseConstraintForce=off  SenseConstraintForceX=off  SenseConstraintForceY=off  SenseConstraintForceZ=off  SenseConstraintTorque=off  SenseConstraintTorqueX=off  SenseConstraintTorqueY=off  SenseConstraintTorqueZ=off  SenseTotalForce=off  SenseTotalForceX=off  SenseTotalForceY=off  SenseTotalForceZ=off  SenseTotalTorque=off  SenseTotalTorqueX=off  SenseTotalTorqueY=off  SenseTotalTorqueZ=off  CompositeWrenchDir=FollowerOnBase  CompositeWrenchFrame=BaseFrame
  B : PMIOPort  Side=Left
  T_knee : PMIOPort  Port=2  Side=Left
  q_knee_FL : PMIOPort  Port=3  Side=Left
  dq_knee_FL : PMIOPort  Port=4  Side=Left
  G : PMIOPort  Port=5  Side=Right
  FL_Foot_Frame : PMIOPort  Port=6  Side=Right
  connections:
  FL_calf_joint/LConn1 -- B/RConn1
  FL_calf/RConn1 -- FL_foot_fixed/LConn1
  FL_calf/LConn1 -- FL_calf_joint/RConn1
  FL_foot/LConn1 -- FL_foot_fixed/RConn1
  G/RConn1 -- FL_foot/RConn1
  T_knee/RConn1 -- FL_calf_joint/LConn2
  FL_calf_joint/RConn2 -- q_knee_FL/RConn1
  FL_calf_joint/RConn3 -- dq_knee_FL/RConn1
  FL_foot/RConn2 -- FL_Foot_Frame/RConn1

== system FinalProjectSimulinkModel_OBSTACLE/Front Left Leg/Front Left Thigh ==
  FL_thigh : Subsystem
  FL_thigh_joint : sm_lib/Joints/Revolute Joint  JointMode=Normal  SenseConstraintForce=off  SenseConstraintForceX=off  SenseConstraintForceY=off  SenseConstraintForceZ=off  SenseConstraintTorque=off  SenseConstraintTorqueX=off  SenseConstraintTorqueY=off  SenseConstraintTorqueZ=off  SenseTotalForce=off  SenseTotalForceX=off  SenseTotalForceY=off  SenseTotalForceZ=off  SenseTotalTorque=off  SenseTotalTorqueX=off  SenseTotalTorqueY=off  SenseTotalTorqueZ=off  CompositeWrenchDir=FollowerOnBase  CompositeWrenchFrame=BaseFrame  EquilibriumPosition=0  EquilibriumPositionUnits=deg  SpringStiffness=0  SpringStiffnessUnits=N*m/deg  DampingCoefficient=0.01  DampingCoefficientUnits=kg*m^2/(rad*s)  TorqueActuationMode=InputTorque  MotionActuationMode=ComputedMotion  SensePosition=on  SenseVelocity=on  SenseAcceleration=off  SenseTorqueForce=off  SenseLowerLimitTorqueForce=off  SenseUpperLimitTorqueForce=off  LowerLimitSpecify=on  LowerLimitBound=-1.0471975512  LowerLimitBoundUnits=rad  LowerLimitStiffness=1e4  LowerLimitStiffnessUnits=N*m/deg  LowerLimitDamping=10  LowerLimitDampingUnits=N*m/(deg/s)  LowerLimitTransitionRegionWidth=0.1  LowerLimitTransitionRegionWidthUnits=deg  UpperLimitSpecify=on  UpperLimitBound=4.18879020479  UpperLimitBoundUnits=rad  UpperLimitStiffness=1e4  UpperLimitStiffnessUnits=N*m/deg  UpperLimitDamping=10  UpperLimitDampingUnits=N*m/(deg/s)  UpperLimitTransitionRegionWidth=0.1  UpperLimitTransitionRegionWidthUnits=deg  PositionTargetSpecify=on  PositionTargetPriority=High  PositionTargetValue=q_hip_pitch_i  PositionTargetValueUnits=rad  VelocityTargetSpecify=off  VelocityTargetPriority=High  VelocityTargetValue=0  VelocityTargetValueUnits=deg/s
  B : PMIOPort  Side=Left
  T_hip_pitch : PMIOPort  Port=2  Side=Left
  q_hip_pitch_FL : PMIOPort  Port=3  Side=Left
  dq_hip_pitch_FL : PMIOPort  Port=4  Side=Left
  F : PMIOPort  Port=5  Side=Right
  connections:
  B/RConn1 -- FL_thigh_joint/LConn1
  FL_thigh/LConn1 -- FL_thigh_joint/RConn1
  F/RConn1 -- FL_thigh/RConn1
  T_hip_pitch/RConn1 -- FL_thigh_joint/LConn2
  FL_thigh_joint/RConn2 -- q_hip_pitch_FL/RConn1
  FL_thigh_joint/RConn3 -- dq_hip_pitch_FL/RConn1

== system FinalProjectSimulinkModel_OBSTACLE/Front Left Leg/Front Left Hip ==
  FL_hip : Subsystem
  FL_hip_joint : sm_lib/Joints/Revolute Joint  JointMode=Normal  SenseConstraintForce=off  SenseConstraintForceX=off  SenseConstraintForceY=off  SenseConstraintForceZ=off  SenseConstraintTorque=off  SenseConstraintTorqueX=off  SenseConstraintTorqueY=off  SenseConstraintTorqueZ=off  SenseTotalForce=off  SenseTotalForceX=off  SenseTotalForceY=off  SenseTotalForceZ=off  SenseTotalTorque=off  SenseTotalTorqueX=off  SenseTotalTorqueY=off  SenseTotalTorqueZ=off  CompositeWrenchDir=FollowerOnBase  CompositeWrenchFrame=BaseFrame  EquilibriumPosition=0  EquilibriumPositionUnits=deg  SpringStiffness=0  SpringStiffnessUnits=N*m/deg  DampingCoefficient=0.01  DampingCoefficientUnits=kg*m^2/(rad*s)  TorqueActuationMode=InputTorque  MotionActuationMode=ComputedMotion  SensePosition=on  SenseVelocity=on  SenseAcceleration=off  SenseTorqueForce=off  SenseLowerLimitTorqueForce=off  SenseUpperLimitTorqueForce=off  LowerLimitSpecify=on  LowerLimitBound=-0.802851455917  LowerLimitBoundUnits=rad  LowerLimitStiffness=1e4  LowerLimitStiffnessUnits=N*m/deg  LowerLimitDamping=10  LowerLimitDampingUnits=N*m/(deg/s)  LowerLimitTransitionRegionWidth=0.1  LowerLimitTransitionRegionWidthUnits=deg  UpperLimitSpecify=on  UpperLimitBound=0.802851455917  UpperLimitBoundUnits=rad  UpperLimitStiffness=1e4  UpperLimitStiffnessUnits=N*m/deg  UpperLimitDamping=10  UpperLimitDampingUnits=N*m/(deg/s)  UpperLimitTransitionRegionWidth=0.1  UpperLimitTransitionRegionWidthUnits=deg  PositionTargetSpecify=on  PositionTargetPriority=High  PositionTargetValue=q_hip_roll_i  PositionTargetValueUnits=rad  VelocityTargetSpecify=off  VelocityTargetPriority=High  VelocityTargetValue=0  VelocityTargetValueUnits=deg/s
  Front Left Hip Fixed : Subsystem
  B : PMIOPort  Side=Left
  T_hip_roll : PMIOPort  Port=2  Side=Left
  q_hip_roll_FL : PMIOPort  Port=3  Side=Left
  dq_hip_roll_FL : PMIOPort  Port=4  Side=Left
  F : PMIOPort  Port=5  Side=Right
  connections:
  FL_hip/LConn1 -- FL_hip_joint/RConn1
  FL_hip/RConn1 -- F/RConn1
  FL_hip/RConn2 -- Front Left Hip Fixed/LConn1
  FL_hip_joint/LConn1 -- B/RConn1
  T_hip_roll/RConn1 -- FL_hip_joint/LConn2
  FL_hip_joint/RConn2 -- q_hip_roll_FL/RConn1
  FL_hip_joint/RConn3 -- dq_hip_roll_FL/RConn1

== system FinalProjectSimulinkModel_OBSTACLE/Front Right Leg/Front Right Calf and Foot ==
  FR_calf : Subsystem
  FR_calf_joint : sm_lib/Joints/Revolute Joint  JointMode=Normal  SenseConstraintForce=off  SenseConstraintForceX=off  SenseConstraintForceY=off  SenseConstraintForceZ=off  SenseConstraintTorque=off  SenseConstraintTorqueX=off  SenseConstraintTorqueY=off  SenseConstraintTorqueZ=off  SenseTotalForce=off  SenseTotalForceX=off  SenseTotalForceY=off  SenseTotalForceZ=off  SenseTotalTorque=off  SenseTotalTorqueX=off  SenseTotalTorqueY=off  SenseTotalTorqueZ=off  CompositeWrenchDir=FollowerOnBase  CompositeWrenchFrame=BaseFrame  EquilibriumPosition=0  EquilibriumPositionUnits=deg  SpringStiffness=0  SpringStiffnessUnits=N*m/deg  DampingCoefficient=0.01  DampingCoefficientUnits=kg*m^2/(rad*s)  TorqueActuationMode=InputTorque  MotionActuationMode=ComputedMotion  SensePosition=on  SenseVelocity=on  SenseAcceleration=off  SenseTorqueForce=off  SenseLowerLimitTorqueForce=off  SenseUpperLimitTorqueForce=off  LowerLimitSpecify=on  LowerLimitBound=-2.69653369433  LowerLimitBoundUnits=rad  LowerLimitStiffness=1e4  LowerLimitStiffnessUnits=N*m/deg  LowerLimitDamping=10  LowerLimitDampingUnits=N*m/(deg/s)  LowerLimitTransitionRegionWidth=0.1  LowerLimitTransitionRegionWidthUnits=deg  UpperLimitSpecify=on  UpperLimitBound=-0.916297857297  UpperLimitBoundUnits=rad  UpperLimitStiffness=1e4  UpperLimitStiffnessUnits=N*m/deg  UpperLimitDamping=10  UpperLimitDampingUnits=N*m/(deg/s)  UpperLimitTransitionRegionWidth=0.1  UpperLimitTransitionRegionWidthUnits=deg  PositionTargetSpecify=on  PositionTargetPriority=High  PositionTargetValue=q_knee_i  PositionTargetValueUnits=rad  VelocityTargetSpecify=off  VelocityTargetPriority=High  VelocityTargetValue=0  VelocityTargetValueUnits=deg/s
  FR_foot : Subsystem
  FR_foot_fixed : sm_lib/Joints/Weld Joint  JointMode=Normal  SenseConstraintForce=off  SenseConstraintForceX=off  SenseConstraintForceY=off  SenseConstraintForceZ=off  SenseConstraintTorque=off  SenseConstraintTorqueX=off  SenseConstraintTorqueY=off  SenseConstraintTorqueZ=off  SenseTotalForce=off  SenseTotalForceX=off  SenseTotalForceY=off  SenseTotalForceZ=off  SenseTotalTorque=off  SenseTotalTorqueX=off  SenseTotalTorqueY=off  SenseTotalTorqueZ=off  CompositeWrenchDir=FollowerOnBase  CompositeWrenchFrame=BaseFrame
  F : PMIOPort  Side=Left
  T_knee : PMIOPort  Port=2  Side=Left
  q_knee_FR : PMIOPort  Port=3  Side=Left
  dq_knee_FR : PMIOPort  Port=4  Side=Left
  G : PMIOPort  Port=5  Side=Right
  FR_Foot_Frame : PMIOPort  Port=6  Side=Right
  connections:
  FR_foot/LConn1 -- FR_foot_fixed/RConn1
  FR_calf_joint/LConn1 -- F/RConn1
  FR_calf/RConn1 -- FR_foot_fixed/LConn1
  FR_calf/LConn1 -- FR_calf_joint/RConn1
  G/RConn1 -- FR_foot/RConn1
  T_knee/RConn1 -- FR_calf_joint/LConn2
  FR_calf_joint/RConn2 -- q_knee_FR/RConn1
  FR_calf_joint/RConn3 -- dq_knee_FR/RConn1
  FR_foot/RConn2 -- FR_Foot_Frame/RConn1

== system FinalProjectSimulinkModel_OBSTACLE/Front Right Leg/Front Right Thigh ==
  FR_thigh : Subsystem
  FR_thigh_joint : sm_lib/Joints/Revolute Joint  JointMode=Normal  SenseConstraintForce=off  SenseConstraintForceX=off  SenseConstraintForceY=off  SenseConstraintForceZ=off  SenseConstraintTorque=off  SenseConstraintTorqueX=off  SenseConstraintTorqueY=off  SenseConstraintTorqueZ=off  SenseTotalForce=off  SenseTotalForceX=off  SenseTotalForceY=off  SenseTotalForceZ=off  SenseTotalTorque=off  SenseTotalTorqueX=off  SenseTotalTorqueY=off  SenseTotalTorqueZ=off  CompositeWrenchDir=FollowerOnBase  CompositeWrenchFrame=BaseFrame  EquilibriumPosition=0  EquilibriumPositionUnits=deg  SpringStiffness=0  SpringStiffnessUnits=N*m/deg  DampingCoefficient=0.01  DampingCoefficientUnits=kg*m^2/(rad*s)  TorqueActuationMode=InputTorque  MotionActuationMode=ComputedMotion  SensePosition=on  SenseVelocity=on  SenseAcceleration=off  SenseTorqueForce=off  SenseLowerLimitTorqueForce=off  SenseUpperLimitTorqueForce=off  LowerLimitSpecify=on  LowerLimitBound=-1.0471975512  LowerLimitBoundUnits=rad  LowerLimitStiffness=1e4  LowerLimitStiffnessUnits=N*m/deg  LowerLimitDamping=10  LowerLimitDampingUnits=N*m/(deg/s)  LowerLimitTransitionRegionWidth=0.1  LowerLimitTransitionRegionWidthUnits=deg  UpperLimitSpecify=on  UpperLimitBound=4.18879020479  UpperLimitBoundUnits=rad  UpperLimitStiffness=1e4  UpperLimitStiffnessUnits=N*m/deg  UpperLimitDamping=10  UpperLimitDampingUnits=N*m/(deg/s)  UpperLimitTransitionRegionWidth=0.1  UpperLimitTransitionRegionWidthUnits=deg  PositionTargetSpecify=on  PositionTargetPriority=High  PositionTargetValue=q_hip_pitch_i  PositionTargetValueUnits=rad  VelocityTargetSpecify=off  VelocityTargetPriority=High  VelocityTargetValue=0  VelocityTargetValueUnits=deg/s
  B : PMIOPort  Side=Left
  T_hip_pitch : PMIOPort  Port=2  Side=Left
  q_hip_pitch_FR : PMIOPort  Port=3  Side=Left
  dq_hip_pitch_FR : PMIOPort  Port=4  Side=Left
  F : PMIOPort  Port=5  Side=Right
  connections:
  F/RConn1 -- FR_thigh/RConn1
  FR_thigh/LConn1 -- FR_thigh_joint/RConn1
  B/RConn1 -- FR_thigh_joint/LConn1
  T_hip_pitch/RConn1 -- FR_thigh_joint/LConn2
  q_hip_pitch_FR/RConn1 -- FR_thigh_joint/RConn2
  dq_hip_pitch_FR/RConn1 -- FR_thigh_joint/RConn3

== system FinalProjectSimulinkModel_OBSTACLE/Front Right Leg/Front Right Hip ==
  FR_hip : Subsystem
  FR_hip_joint : sm_lib/Joints/Revolute Joint  JointMode=Normal  SenseConstraintForce=off  SenseConstraintForceX=off  SenseConstraintForceY=off  SenseConstraintForceZ=off  SenseConstraintTorque=off  SenseConstraintTorqueX=off  SenseConstraintTorqueY=off  SenseConstraintTorqueZ=off  SenseTotalForce=off  SenseTotalForceX=off  SenseTotalForceY=off  SenseTotalForceZ=off  SenseTotalTorque=off  SenseTotalTorqueX=off  SenseTotalTorqueY=off  SenseTotalTorqueZ=off  CompositeWrenchDir=FollowerOnBase  CompositeWrenchFrame=BaseFrame  EquilibriumPosition=0  EquilibriumPositionUnits=deg  SpringStiffness=0  SpringStiffnessUnits=N*m/deg  DampingCoefficient=0.01  DampingCoefficientUnits=kg*m^2/(rad*s)  TorqueActuationMode=InputTorque  MotionActuationMode=ComputedMotion  SensePosition=on  SenseVelocity=on  SenseAcceleration=off  SenseTorqueForce=off  SenseLowerLimitTorqueForce=off  SenseUpperLimitTorqueForce=off  LowerLimitSpecify=on  LowerLimitBound=-0.802851455917  LowerLimitBoundUnits=rad  LowerLimitStiffness=1e4  LowerLimitStiffnessUnits=N*m/deg  LowerLimitDamping=10  LowerLimitDampingUnits=N*m/(deg/s)  LowerLimitTransitionRegionWidth=0.1  LowerLimitTransitionRegionWidthUnits=deg  UpperLimitSpecify=on  UpperLimitBound=0.802851455917  UpperLimitBoundUnits=rad  UpperLimitStiffness=1e4  UpperLimitStiffnessUnits=N*m/deg  UpperLimitDamping=10  UpperLimitDampingUnits=N*m/(deg/s)  UpperLimitTransitionRegionWidth=0.1  UpperLimitTransitionRegionWidthUnits=deg  PositionTargetSpecify=on  PositionTargetPriority=High  PositionTargetValue=-q_hip_roll_i  PositionTargetValueUnits=rad  VelocityTargetSpecify=off  VelocityTargetPriority=High  VelocityTargetValue=0  VelocityTargetValueUnits=deg/s
  Front Right Hip Fixed : Subsystem
  B : PMIOPort  Side=Left
  T_hip_roll : PMIOPort  Port=2  Side=Left
  q_hip_roll_FR : PMIOPort  Port=3  Side=Left
  dq_hip_roll_FR : PMIOPort  Port=4  Side=Left
  F : PMIOPort  Port=5  Side=Right
  connections:
  FR_hip/LConn1 -- FR_hip_joint/RConn1
  FR_hip/RConn1 -- F/RConn1
  FR_hip/RConn2 -- Front Right Hip Fixed/LConn1
  FR_hip_joint/LConn1 -- B/RConn1
  T_hip_roll/RConn1 -- FR_hip_joint/LConn2
  FR_hip_joint/RConn2 -- q_hip_roll_FR/RConn1
  FR_hip_joint/RConn3 -- dq_hip_roll_FR/RConn1
